simulink model "PFC_IBC_AC_Model"  (R2025a)
settings: Solver=VariableStepAuto  StartTime=0.0  StopTime=0.1  RelTol=1e-3
undefined symbols (not defined in the file): D_val, fp_val, L_val, RL_val, Vin_peak_val
libraries: spsSeriesRLCBranchLib x4, spsDiodeLib x2, spsMosfetLib x2, spsVoltageMeasurementLib x2, spsACVoltageSourceLib x1, spsCurrentMeasurementLib x1, spsUniversalBridgeLib x1, spspowerguiLib x1
settings Model: Creator=rohan  LastModifiedBy=rohan
settings SolverCC: ZeroCrossControl=DisableAll

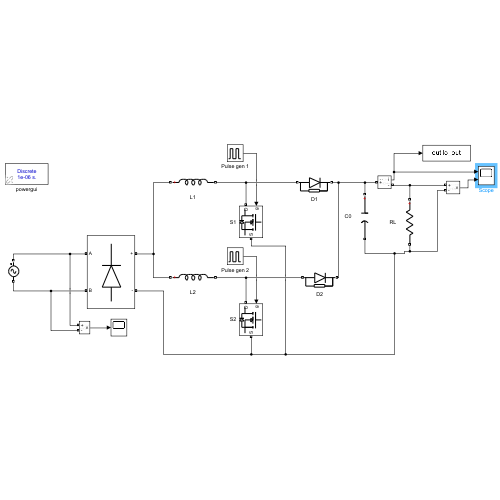
[thumbnail: Simulink's stored preview of the top-level diagram]
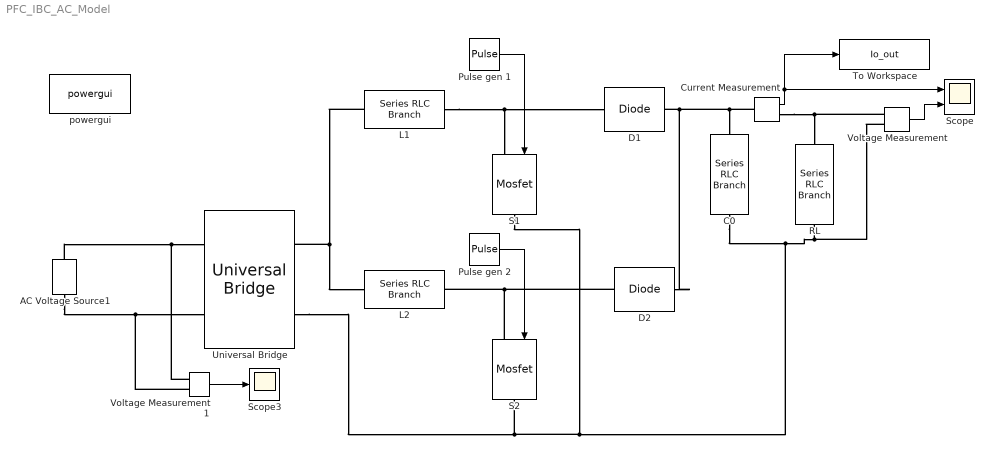
== system PFC_IBC_AC_Model ==
  AC Voltage Source1 : spsACVoltageSourceLib/AC Voltage Source  Amplitude=Vin_peak_val  Phase=0  Frequency=50  SampleTime=0  Measurements=None  BusType=swing  Pref=10e3  Qref=0  Qmin=-inf  Qmax=+inf
  C0 : spsSeriesRLCBranchLib/Series RLC Branch  LConnTagsString=__new0  RConnTagsString=__new0  BranchType=C  Resistance=1  Inductance=1e-3  SetiL0=off  InitialCurrent=0  Capacitance=470e-6  Setx0=off  InitialVoltage=0  Measurements=None
  Current Measurement : spsCurrentMeasurementLib/Current Measurement  PhasorSimulation=off  OutputType=Complex  PSBequivalent=0
  D1 : spsDiodeLib/Diode  Ron=0.001  Lon=0  Vf=0.8  IC=0  UseSnubber=0  Rs=500  Cs=250e-9  Measurements=off
  D2 : spsDiodeLib/Diode  Ron=0.001  Lon=0  Vf=0.8  IC=0  UseSnubber=0  Rs=500  Cs=250e-9  Measurements=off
  L1 : spsSeriesRLCBranchLib/Series RLC Branch  LConnTagsString=__new0  RConnTagsString=__new0  BranchType=L  Resistance=1  Inductance=L_val  SetiL0=off  InitialCurrent=0  Capacitance=1e-6  Setx0=off  InitialVoltage=0  Measurements=None
  L2 : spsSeriesRLCBranchLib/Series RLC Branch  LConnTagsString=__new0  RConnTagsString=__new0  BranchType=L  Resistance=1  Inductance=L_val  SetiL0=off  InitialCurrent=0  Capacitance=1e-6  Setx0=off  InitialVoltage=0  Measurements=None
  "Pulse gen 1 " : DiscretePulseGenerator  PulseType=Time based  Period=1/fp_val  PulseWidth=D_val
  Pulse gen 2 : DiscretePulseGenerator  PulseType=Time based  Period=1/fp_val  PulseWidth=D_val  PhaseDelay=(1/fp_val)/2
  RL : spsSeriesRLCBranchLib/Series RLC Branch  LConnTagsString=__new0  RConnTagsString=__new0  BranchType=R  Resistance=RL_val  Inductance=1e-3  SetiL0=off  InitialCurrent=0  Capacitance=1e-6  Setx0=off  InitialVoltage=0  Measurements=None
  S1 : spsMosfetLib/Mosfet  Ron=0.1  Lon=0  Rd=0.01  Vfd=0  IC=0  Rs=1e5  Cs=inf  Measurements=off
  S2 : spsMosfetLib/Mosfet  Ron=0.1  Lon=0  Rd=0.01  Vfd=0  IC=0  Rs=1e5  Cs=inf  Measurements=off
  Scope : Scope  NumInputPorts=2
      settings: ActiveDisplayYMinimum=-0.96184757090130013  ActiveDisplayYMaximum=5.7358734046012394
  Scope3 : Scope
      settings: ActiveDisplayYMinimum=-386.59108448021021  ActiveDisplayYMaximum=386.59108448021021  DataLoggingVariableName=ScopeData3
  To Workspace : ToWorkspace  VariableName=Io_out  SaveFormat=Timeseries  SampleTime=-1
  Universal Bridge : spsUniversalBridgeLib/Universal Bridge  Arms=2  SnubberResistance=1e5  SnubberCapacitance=inf  Device=Diodes  Ron=1e-3  Lon=0  ForwardVoltages="[  0  0  ]"  ForwardVoltage=0  GTOparameters=[ 10e-6 , 20e-6 ]  IGBTparameters=[ 1e-6 , 2e-6 ]  Measurements=None  Measurements_2=None  converterType=Rectifier
  Voltage Measurement : spsVoltageMeasurementLib/Voltage Measurement  PhasorSimulation=off  OutputType=Complex  PSBequivalent=0
  Voltage Measurement1 : spsVoltageMeasurementLib/Voltage Measurement  PhasorSimulation=off  OutputType=Complex  PSBequivalent=0
  powergui : spspowerguiLib/powergui  Priority=1  SimulationMode=Discrete  SampleTime=1e-6  frequency=60  Iterations=50  frequencyindice=50  Pbase=100e6  ErrMax=1e-4  UnitsV=kV  UnitsW=MW  buscounter=0  FunctionMessages=off  echomessages=off  EnableUseOfTLC=off  CurrentSourceSwitches=off  DisableSnubberDevices=off  DisableRonSwitches=off  DisableVfSwitches=off  DisplayEquations=off  AutomaticDiscreteSolvers=off  SolverType=Tustin/Backward Euler (TBE)  Interpol=off  ExternalGateDelay=off  methode=off  Ts=100  x0status=blocks  SPID=on  SwTol=0  HookPort=off  NonlinearTolerance=1e-4  nMaxIteration=100  ContinueOnMaxIteration=off  RestoreLinks=warning  ResistiveCurrentMeasurement=off  Frange=[0:2:500]  Ylog=off  Xlog=on  ShowGrid=off  save=off  variable=ZData  structure=0  ZoomFFT=off  StartTime=0.0  cycles=1  DisplayStyle=1  fundamental=60  FreqAxis=off  MaxFrequency=1000  frequencyindicesteady=1  RmsSteady=1  display=off
  wires:
  Current Measurement/1 -> To Workspace/1, Scope/1
  Voltage Measurement/1 -> Scope/2
  "Pulse gen 1 "/1 -> S1/1
  Pulse gen 2/1 -> S2/1
  Voltage Measurement1/1 -> Scope3/1
  connections:
  AC Voltage Source1/LConn1 -- Voltage Measurement1/LConn2 -- Universal Bridge/LConn2
  L1/LConn1 -- L2/LConn1 -- Universal Bridge/RConn1
  D2/LConn1 -- S2/LConn1 -- L2/RConn1
  Current Measurement/LConn1 -- C0/LConn1 -- D2/RConn1 -- D1/RConn1
  S1/RConn1 -- Voltage Measurement/LConn2 -- RL/RConn1 -- C0/RConn1 -- S2/RConn1 -- Universal Bridge/RConn2
  L1/RConn1 -- S1/LConn1 -- D1/LConn1
  Current Measurement/RConn1 -- Voltage Measurement/LConn1 -- RL/LConn1
  AC Voltage Source1/RConn1 -- Voltage Measurement1/LConn1 -- Universal Bridge/LConn1
